simulink model "elevation_lin"  (R2017b)
settings: Solver=VariableStepAuto  StartTime=0.0  StopTime=10.0  RelTol=1e-3
values from neighbouring files (symbols this model uses):
  aetop = .8494    (= 0.8494)    [Sim_Constants.m]
  cdrag = 1.3    [Sim_Constants.m]
  dair = 1.225    [Sim_Constants.m]
  g = 9.8    [Sim_Constants.m]    (also in startup.m)
  m = 3.65    [Sim_Constants.m]    (also in startup.m)
libraries: simulink x1, simulink_extras x1
settings Model: Creator=schapman  LastModifiedBy=DanAdmin

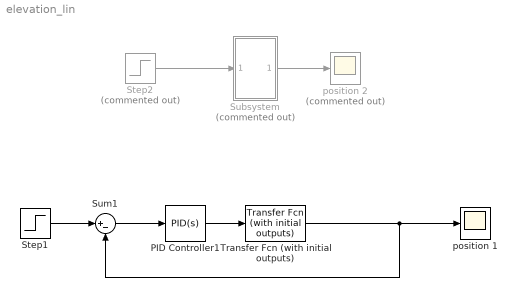
== system elevation_lin ==
  PID Controller1 : simulink/Continuous/PID Controller  Controller=PID  TimeDomain=Continuous-time  SampleTime=-1  IntegratorMethod=Forward Euler  FilterMethod=Forward Euler  Form=Parallel  UseFilter=on  ControllerParametersSource=internal  P=1.66191966416835  I=0.241181379439698  D=2.85661577707218  N=361.393937805181  InitialConditionSource=internal  InitialConditionForIntegrator=0  InitialConditionForFilter=0  ExternalReset=none  LimitOutput=off  UpperSaturationLimit=inf  LowerSaturationLimit=-inf  LinearizeAsGain=on  AntiWindupMode=none  Kb=1  TrackingMode=off  Kt=1  PParamMin=[]  PParamMax=[]  IParamMin=[]  IParamMax=[]  DParamMin=[]  DParamMax=[]  NParamMin=[]  NParamMax=[]  KbParamMin=[]  KbParamMax=[]  KtParamMin=[]  KtParamMax=[]  POutMin=[]  POutMax=[]  IOutMin=[]  IOutMax=[]  DOutMin=[]  DOutMax=[]  NOutMin=[]  NOutMax=[]  KbOutMin=[]  KbOutMax=[]  KtOutMin=[]  KtOutMax=[]  IntegratorOutMin=[]  IntegratorOutMax=[]  FilterOutMin=[]  FilterOutMax=[]  SumOutMin=[]  SumOutMax=[]  SumI1OutMin=[]  SumI1OutMax=[]  SumI2OutMin=[]  SumI2OutMax=[]  SumI3OutMin=[]  SumI3OutMax=[]  SumDOutMin=[]  SumDOutMax=[]  SaturationOutMin=[]  SaturationOutMax=[]  IntegratorContinuousStateAttributes=''  IntegratorStateMustResolveToSignalObject=off  IntegratorRTWStateStorageClass=Auto  FilterContinuousStateAttributes=''  FilterStateMustResolveToSignalObject=off  FilterRTWStateStorageClass=Auto  DifferentiatorICPrevScaledInput=0  DifferentiatorOutMin=[]  DifferentiatorOutMax=[]  InitialConditionSetting=State (most efficient)  FilterDiffOutCoefMin=[]  FilterDiffOutCoefMax=[]  SumDenOutMin=[]  SumDenOutMax=[]  SumNumOutMin=[]  SumNumOutMax=[]  ReciprocalOutMin=[]  ReciprocalOutMax=[]  DivideOutMin=[]  DivideOutMax=[]  TunerSelectOption=Transfer Function Based (PID Tuner App)
  Step1 : Step  Time=2  After=10  SampleTime=0
  Step2 : Step  Commented=on  Time=2  After=10  SampleTime=0
  Subsystem : Subsystem  Commented=on
  Sum1 : Sum  Inputs=|+-
  Transfer Fcn (with initial outputs) : simulink_extras/Additional Linear/Transfer Fcn (with initial outputs)  N=[1.096]  D="[1  0 0]"  Y0=0  U0=0
  position 1 : Scope
  position 2 : Scope  Commented=on
  wires:
  Transfer Fcn (with initial outputs)/1 -> Sum1/2, position 1/1
  Step1/1 -> Sum1/1
  Sum1/1 -> PID Controller1/1
  PID Controller1/1 -> Transfer Fcn (with initial outputs)/1
  Step2/1 -> Subsystem/1(In1)
  Subsystem/1(Out1) -> position 2/1

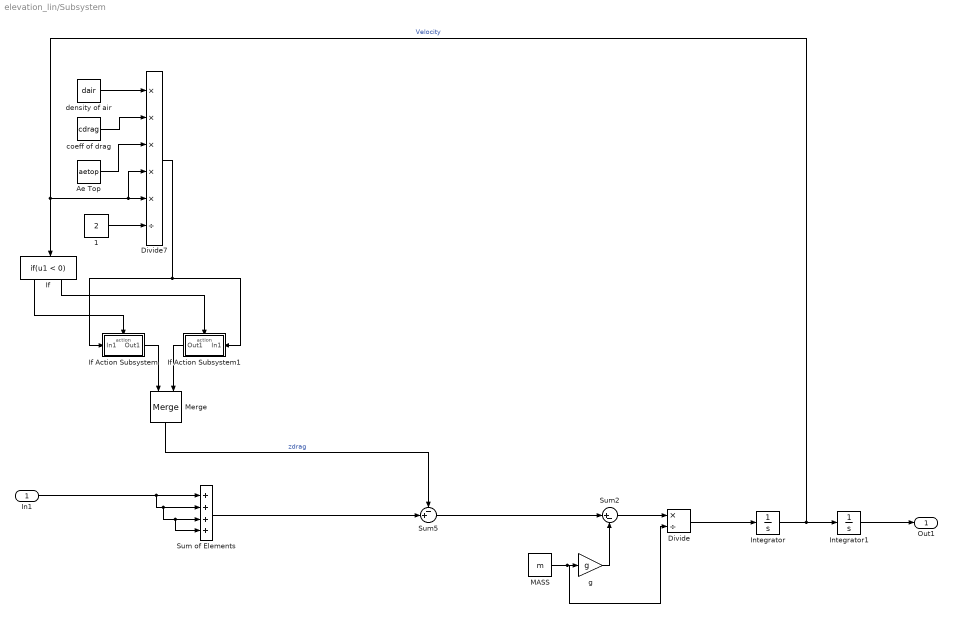
== system elevation_lin/Subsystem ==
  In1 : Inport
  1 : Constant  Value=2
  Ae Top : Constant  Value=aetop
  Divide : Product  Inputs=*/
  Divide7 : Product  Inputs=*****/
  If : If  IfExpression=u1 < 0
  If Action Subsystem : Subsystem  TreatAsAtomicUnit=on
  If Action Subsystem1 : Subsystem  TreatAsAtomicUnit=on
  Integrator : Integrator
  Integrator1 : Integrator
  MASS : Constant  Value=m
  Merge : Merge
  Sum of Elements : Sum  Inputs=++++
  Sum2 : Sum  Inputs=|+-
  Sum5 : Sum  Inputs=-+|
  coeff of drag : Constant  Value=cdrag
  density of air : Constant  Value=dair
  g : Gain  Gain=g
  Out1 : Outport
  wires:
  Divide7/1 -> If Action Subsystem/1(In1), If Action Subsystem1/1(In1)
  If/2 -> If Action Subsystem1/Action
  If Action Subsystem/1(Out1) -> Merge/1
  coeff of drag/1 -> Divide7/2
  Merge/1 -> Sum5/1  "zdrag"
  If/1 -> If Action Subsystem/Action
  Integrator/1 -> Integrator1/1, Divide7/4, Divide7/5, If/1  "Velocity"
  If Action Subsystem1/1(Out1) -> Merge/2
  Ae Top/1 -> Divide7/3
  1/1 -> Divide7/6
  density of air/1 -> Divide7/1
  Divide/1 -> Integrator/1
  Sum2/1 -> Divide/1
  Sum5/1 -> Sum2/1
  g/1 -> Sum2/2
  MASS/1 -> Divide/2, g/1
  Sum of Elements/1 -> Sum5/2
  In1/1 -> Sum of Elements/4, Sum of Elements/3, Sum of Elements/2, Sum of Elements/1
  Integrator1/1 -> Out1/1

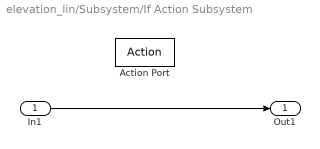
== system elevation_lin/Subsystem/If Action Subsystem ==
  In1 : Inport
  Action Port : ActionPort  ActionType=then
  Out1 : Outport
  wires:
  In1/1 -> Out1/1

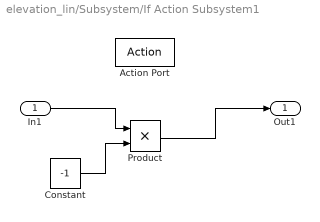
== system elevation_lin/Subsystem/If Action Subsystem1 ==
  In1 : Inport
  Action Port : ActionPort  ActionType=else
  Constant : Constant  Value=-1
  Product : Product
  Out1 : Outport
  wires:
  In1/1 -> Product/1
  Constant/1 -> Product/2
  Product/1 -> Out1/1
